simulink library "sphero_lib"  (Simulink 8.8)
settings: Solver=ode45  StartTime=0.0  StopTime=10.0  RelTol=1e-3
libraries: simulink x2
settings Model: Creator=gvallabh  LastModifiedBy=gcampa

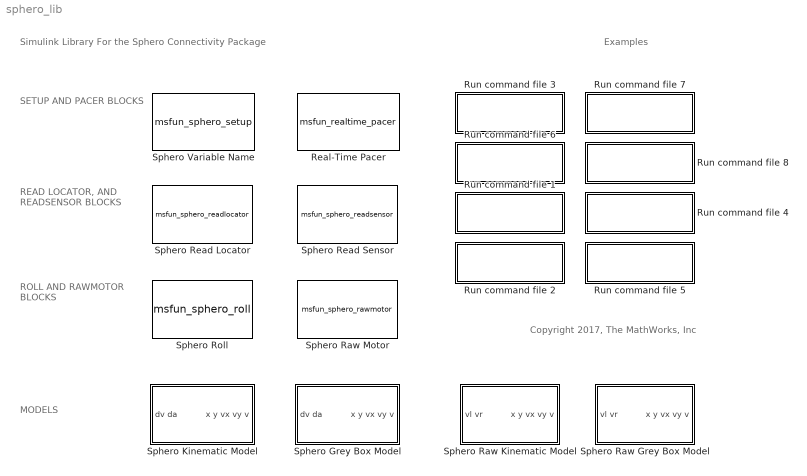
== system sphero_lib ==
  note: Copyright 2017, The MathWorks, Inc
  note: SETUP
      | AND PACER
      | BLOCKS
  note: Simulink Library For the Sphero Connectivity Package
  note: READ LOCATOR,
      | AND READSENSOR
      | BLOCKS
  note: Examples
  note: ROLL AND
      | RAWMOTOR
      | BLOCKS
  note: MODELS
  Real-Time Pacer : M-S-Function  FunctionName=msfun_realtime_pacer  Parameters=simTimePerRealTime  mask(RealTime_Pacer){simTimePerRealTime=1}
      mask prompts: simTimePerRealTime "Speedup (Simulation Time / Real Time):"
      mask help:
      | Slow down a simulation to track real (i.e., wall clock) elapsed time.
      |
      | "Speedup" specifies the ratio between simulation time and real time
      |  Speedup = N => N sec. of simulation time per sec. of real time
      |  Speedup can be fractional (e.g., 0.5, 1.3).
      |  Speedup = inf => allow simulation to run at full speed
      |
      | Click on the Help button for details.
      mask Help: web('realtime_pacer_help.html', '-helpbrowser')
      mask Display: fprintf('Real-Time Pacer\nSpeedup = %g', simTimePerRealTime)
  Run command file 1 : Subsystem
      settings: OpenFcn=rawmotor_sim
      mask Display: disp('Command \nRaw Motors')
  Run command file 2 : Subsystem
      settings: OpenFcn=sph_control_sim
      mask Display: disp('Control \nExample')
  Run command file 3 : Subsystem
      settings: OpenFcn=accel_sim
      mask Display: disp('Read Sensor \n (Acceleration)')
  Run command file 4 : Subsystem
      settings: OpenFcn=rawmotor_sim_kine
      mask Display: disp('Raw Kinematic Model\n Open Loop')
  Run command file 5 : Subsystem
      settings: OpenFcn=rawmotor_sim_grey
      mask Display: disp('Raw Grey Box Model\n Open Loop')
  Run command file 6 : Subsystem
      settings: OpenFcn=roll_sim
      mask Display: disp('Roll and\n Read Location')
  Run command file 7 : Subsystem
      settings: OpenFcn=sph_control_sim_kine
      mask Display: disp('Kinematic Model\n Control')
  Run command file 8 : Subsystem
      settings: OpenFcn=sph_control_sim_grey
      mask Display: disp('Grey Box Model\n Control')
  Sphero Grey Box Model : Subsystem  mask(Sphero Grey Box Model){num=[5.4], den=[1 3.8], vtr=[5 50], vmax=1500, Nva=[1 0.1], D=[1 1], P0=[0 0], T=0.1}
      mask prompts: num "Speed transfer function numerator"; den "Speed transfer function denominator"; vtr "Thresholds for current and desired speed (0 to 255)"; vmax "Maximum speed (mm/s)"; Nva "Input noise powers for desired speed and angle"; D "Send and Receive delay lengths"; P0 "Initial Position along x and y (cm)"; T "Sample Time"
      mask help:
      | This block is a grey-box model of the Sphero. The input vector contains the desired speed dv (from 0 to 255) and desired angle da in degrees. The output vector contains 5 elements: the positions along x and y axis (in mm), the velocities along the same axis (in mm/sec), and the total speed, (that is the magnitude of the velocity vector).
      |
      | The kinematics are modeled as an unicycle, that is [xdot ydot]=v*[sin(a) cos(a)] where v and a are speed and angle. The angle a is assumed equal to the desired angle input.
      |
      | The relationship between the speed v and the desired speed input dv is modeled by a continuous time transfer function (active when both the current and desired speed are greater than a given threshold), followed by a rescaling to the range [0 vmax], where vmax is the maximum speed (when dv=255) in mm/s. Noise is inserted at the block input, while transmission delays are used both at the block input and output.
      mask init:
      | x0=P0(1);y0=P0(2);
      mask Help:
      | This block is a grey-box model of the Sphero. The input vector contains the desired speed dv (from 0 to 255) and desired angle da in degrees. The output vector contains 5 elements: the positions along x and y axis (in mm), the velocities along the same axis (in mm/sec), and the total speed, (that is the magnitude of the velocity vector).
      | 
      | The kinematics are modeled as an unicycle, that is [xdot ydot]=v*[sin(a) cos(a)] where v and a are speed and angle. The angle a is assumed equal to the desired angle input.
      | 
      | The relationship between the speed v and the desired speed input dv is modeled by a continuous time transfer function (active when both the current and desired speed are greater than a given threshold), followed by a rescaling to the range [0 vmax], where vmax is the maximum speed (when dv=255) in mm/s. Noise is inserted at the block input, while transmission delays are used both at the block input and output.
      | 
      | Look under the mask for more information.
  Sphero Kinematic Model : Subsystem  mask(Sphero Kinematic Model){vmax=1500, P0=[0 0]}
      mask prompts: vmax "Max Speed (mm/s)"; P0 "Initial Position along x and y (cm)"
      mask help:
      | This block is a pure kinematic model of the Sphero.
      |
      | The input vector contains the desired speed dv (from 0 to 255) and desired angle da in degrees. The output vector contains 5 elements: the positions along x and y axis (in mm), the velocities along the same axis (in mm/sec), and the total speed, (that is the magnitude of the velocity vector).
      |
      | The kinematics are modeled as an unicycle, that is [xdot ydot]=v*[sin(a) cos(a)] where v and a are speed and angle. The angle a is assumed equal to the desired angle input da. The speed v is a rescaling of the input dv from the range [0 255] to the range [0 vmax],  (that is v=vmax/255*dv) where vmax is the maximum speed in mm/s.
      mask init:
      | x0=P0(1);y0=P0(2);
      mask Help:
      | This block is a pure kinematic model of the Sphero.
      | 
      | The input vector contains the desired speed dv (from 0 to 255) and desired angle da in degrees. The output vector contains 5 elements: the positions along x and y axis (in mm), the velocities along the same axis (in mm/sec), and the total speed, (that is the magnitude of the velocity vector).
      | 
      | The kinematics are modeled as an unicycle, that is [xdot ydot]=v*[sin(a) cos(a)] where v and a are speed and angle. The angle a is assumed equal to the desired angle input da. The speed v is a rescaling of the input dv from the range [0 255] to the range [0 vmax],  (that is v=vmax/255*dv) where vmax is the maximum speed in mm/s.
      | 
      | Please look under the mask for further information.
  Sphero Raw Grey Box Model : Subsystem  mask(Sphero Grey Box Model){num_v=[5.4], den_v=[1 3.8], vtr=[5 50], num_w=[0.59], den_w=[1 0.1], vmax=1500, Nvw=[1 0.1]*0, D=[1 1], T=0.1, P0=[0 0]}
      mask prompts: num_v "Speed transfer function numerator"; den_v "Speed transfer function denominator"; vtr "Thresholds for current and desired speed (0 to 255)"; num_w "Angular speed transfer function numerator"; den_w "Angular speed transfer function denominator"; vmax "Maximum speed (mm/s)"; Nvw "Input noise powers for desired speed and angle"; D "Send and Receive delay lengths"; T "Sample Time"; P0 "Initial Position along x and y (cm)"
      mask help:
      | This block is a grey-box model of the Sphero. The input vector contains the desired speed of left and right motors (from 0 to 255). The output vector contains 5 elements: the positions along x and y axis (in mm), the velocities along the same axis (in mm/sec), and the total speed, (that is the magnitude of the velocity vector).
      |
      | The kinematics are modeled as an unicycle, that is [xdot ydot]=v*[sin(a) cos(a)] where v and a are speed and angle. The relationship between the speed v and the speed command (L+R)/2  is modeled by a continuous time transfer function (active when both the current and desired speed are greater than a given threshold), followed by a rescaling to the range [0 vmax], where vmax is the maximum speed (when dv=255) in mm/s. The  relationship between the angle a and the angular speed command (L-R)/2  is modeled by a continuous time transfer function (having static gain equal to wmax/255, where wmax is the maximum angular speed) followed by an integrator. Noise is inserted at the block input, while transmission delays are used both at the block input and output.
      mask init:
      | x0=P0(1);y0=P0(2);
      mask Help:
      | This block is a grey-box model of the Sphero. The input vector contains the desired speed of left and right motors (from 0 to 255). The output vector contains 5 elements: the positions along x and y axis (in mm), the velocities along the same axis (in mm/sec), and the total speed, (that is the magnitude of the velocity vector).
      | 
      | The kinematics are modeled as an unicycle, that is [xdot ydot]=v*[sin(a) cos(a)] where v and a are speed and angle. The relationship between the speed v and the speed command (L+R)/2  is modeled by a continuous time transfer function (active when both the current and desired speed are greater than a given threshold), followed by a rescaling to the range [0 vmax], where vmax is the maximum speed (when dv=255) in mm/s. The  relationship between the angle a and the angular speed command (L-R)/2  is modeled by a continuous time transfer function (having static gain equal to wmax/255, where wmax is the maximum angular speed) followed by an integrator. Noise is inserted at the block input, while transmission delays are used both at the block input and output.
      | 
      | Look under the mask for more information.
  "Sphero Raw Kinematic Model " : Subsystem  mask(Sphero Grey Box Model){vmax=1500, wmax=1500, P0=[0 0]}
      mask prompts: vmax "Maximum speed (mm/s)"; wmax "Maximum angular speed (deg/s)"; P0 "Initial Position along x and y (cm)"
      mask help:
      | This block is a grey-box model of the Sphero. The input vector contains the desired speed of left and right motors (from 0 to 255). The output vector contains 5 elements: the positions along x and y axis (in mm), the velocities along the same axis (in mm/sec), and the total speed, (that is the magnitude of the velocity vector).
      |
      | The kinematics are modeled as an unicycle, that is [xdot ydot]=v*[sin(a) cos(a)] where v and a are speed and angle. The speed v is a rescaling of the the speed input (L+R)/2 from the range [0 255] to the range [0 vmax],  (that is v=vmax/255*(L+R)/2) where vmax is the maximum speed in mm/s. Similarly, the angluar speed w is a rescaling of the the anngular speed input (L-R)/2 from the range [0 255] to the range [0 wmax],  (that is v=wmax/255*(L-R)/2) where wmax is the maximum angular speed in deg/s. The angle a is the integral of the angular speed.
      mask init:
      | x0=P0(1);y0=P0(2);
      mask Help:
      | This block is a grey-box model of the Sphero. The input vector contains the desired speed of left and right motors (from 0 to 255). The output vector contains 5 elements: the positions along x and y axis (in mm), the velocities along the same axis (in mm/sec), and the total speed, (that is the magnitude of the velocity vector).
      | 
      | The kinematics are modeled as an unicycle, that is [xdot ydot]=v*[sin(a) cos(a)] where v and a are speed and angle. The speed v is a rescaling of the the speed input (L+R)/2 from the range [0 255] to the range [0 vmax],  (that is v=vmax/255*(L+R)/2) where vmax is the maximum speed in mm/s. Similarly, the angluar speed w is a rescaling of the the anngular speed input (L-R)/2 from the range [0 255] to the range [0 wmax],  (that is v=wmax/255*(L-R)/2) where wmax is the maximum angular speed in deg/s. The angle a is the integral of the angular speed.
      | 
      | Look under the mask for more information.
  Sphero Raw Motor : M-S-Function  FunctionName=msfun_sphero_rawmotor  Parameters="SpheroVarNumber,  T"  mask(Sphero Raw Motor){SpheroVarNumber=Existing workspace Sphero variable #1, T=0.2}
      mask prompts: SpheroVarNumber "Sphero Variable"; T "Sample Time (-1 for inherited)"
      mask help:
      | Every time this block is executed it gets the 2-elements vector at its input, which contains the power of the left and right motors respectively, and calls the MATLAB "rawMotor" function to move the Sphero motors accordingly. Note that the mode is set to reverse if the specified speed is negative.
      |
      | The first parameter in the mask is the name of the Sphero object (which must match the one chosen in the Setup block). The second parameter is the sample time.
      |
      | See the help for more details.
      mask Help:
      | Every time this block is executed it gets the 2-elements vector at its input, which contains the power of the left and right motors respectively, and calls the MATLAB "rawMotor" function to move the Sphero motors accordingly. Note that the mode is set to reverse if the specified speed is negative.
      | 
      | The first parameter in the mask is the name of the Sphero object (which must match the one chosen in the Setup block). The second parameter is the sample time.
      | 
      | The corresponding Sphero method is "rawMotor", so you can type "doc sphero.rawMotor" or "help sphero.rawMotor" for more details.
      mask TypeOptions SpheroVarNumber: Existing workspace Sphero variable #1 | Existing workspace Sphero variable #2 | Existing workspace Sphero variable #3 | Existing workspace Sphero variable #4
      mask Display:
      | try
      |     SetupBlockName = find_system(bdroot(gcb),'SearchDepth', 1, 'MaskType', 'Sphero Name Setup', 'SpheroVarNumber', SpheroVarNumber);
      |     str=get_param(SetupBlockName,'workspaceVarName');
      |     fprintf('%s\nrawMotor\n',str{1});
      | catch
      |     fprintf('Workspace var #%s\nrawMotor\n',SpheroVarNumber(end))
      | end
      | 
      | color('gray')
      | fprintf('\n\n [left right]');
  Sphero Read Locator : M-S-Function  FunctionName=msfun_sphero_readlocator  Parameters=SpheroVarNumber, T  mask(Sphero Read Locator){SpheroVarNumber=Existing workspace Sphero variable #1, T=0.2}
      mask prompts: SpheroVarNumber "Sphero Variable"; T "Sample Time (-1 for inherited):"
      mask help:
      | Every time this block is executed it calls the MATLAB "readLocator" function, which returns the current location and velocity components of the Sphero.
      |
      | The output of the block is a 5-element vector containing respectively the position along the x and y axes, the velocity along x and y axes, and the speed of the Sphero.
      |
      | The first parameter in the mask is the name of the Sphero object (which must match the one chosen in the Setup block).
      | The second parameter is the sample time.
      |
      | See the help for more details.
      mask Help:
      | Every time this block is executed it calls the MATLAB readLocator function, which returns the current location and velocity components of the Sphero.
      | 
      | The output of the block is a 5-element vector containing respectively the position along the x and y axes, the velocity along x and y axes, and the speed of the Sphero.
      | 
      | All the data received from the sphero are int16 values, which are then casted to doubles at the block output. Specifically, the positions are signed values in cm, velocities are signed in cm/sec, and the speed is unsigned in cm/sec.
      | 
      | The first parameter in the mask is the name of the Sphero object (which must match the one chosen in the Setup block).
      | The second parameter is the sample time.
      | 
      | The corresponding MATLAB command is "readLocator", so you can type "doc sphero.readLocator" or "help sphero.readLocator" for more details.
      mask TypeOptions SpheroVarNumber: Existing workspace Sphero variable #1 | Existing workspace Sphero variable #2 | Existing workspace Sphero variable #3 | Existing workspace Sphero variable #4
      mask Display:
      | try
      |     SetupBlockName = find_system(bdroot(gcb),'SearchDepth', 1, 'MaskType', 'Sphero Name Setup', 'SpheroVarNumber', SpheroVarNumber);
      |     str=get_param(SetupBlockName,'workspaceVarName');
      |     fprintf('%s\nreadLocator\n',str{1});
      | catch
      |     fprintf('Workspace var #%s\nreadLocator\n',SpheroVarNumber(end))
      | end
      | 
      | color('gray')
      | fprintf('\n\n [x  y  vx  vy  v]');
  Sphero Read Sensor : M-S-Function  FunctionName=msfun_sphero_readsensor  Parameters=SpheroVarNumber, SensorString, T  mask(Sphero Read Sensor){SpheroVarNumber=Existing workspace Sphero variable #1, SensorString=accelX, T=1}
      mask prompts: SpheroVarNumber "Sphero Variable"; SensorString "Sensor"; T "Sample Time (-1 for inherited):"
      mask help:
      | Every time this block is executed it calls the MATLAB "readSensor" function, which reads a specified sensor and returns its value.
      |
      | The output of the block is a scalar containing the value measured by the sensor.
      |
      | The first parameter in the mask is the name of the Sphero object (which must match the one chosen in the Setup block).
      | The second parameter is the sensor to be read.
      | The third parameter is the sample time.
      |
      | See the help for more details.
      mask Help:
      | Every time this block is executed it calls the MATLAB "readSensor" function, which reads a specified sensor and returns its value.
      | 
      | The output of the block is a scalar containing the value measured by the sensor.
      | All the data received from the sphero are int16 values, which are then casted to doubles at the block output. Specifically, the positions are signed values in cm, velocities are signed in cm/sec, and the speed is unsigned in cm/sec.
      | 
      | The first parameter in the mask is the name of the Sphero object (which must match the one chosen in the Setup block).
      | 
      | The second parameter is the sensor to be read.It must be one of these strings: 'accelX', 'accelY', 'accelZ', 'gyroX', 'gyroY', 'gyroZ','rmotorEmfRaw', 'lmotorEmfRaw', 'lmotorPwmRaw', 'rmotorPwmRaw','imuPitch', 'imuRoll', 'imuYaw', 'accelXFilt', 'accelYFilt','accelZFilt', 'gyroXFilt', 'gyroYFilt', 'gyroZFilt','rmotorEmfFilt', 'lmotorEmfFilt', 'Q0', 'Q1', 'Q2', 'Q3', 'distX','distY', 'accelOne', 'velX', 'velY'
      | 
      | The third parameter is the sample time.
      mask TypeOptions SpheroVarNumber: Existing workspace Sphero variable #1 | Existing workspace Sphero variable #2 | Existing workspace Sphero variable #3 | Existing workspace Sphero variable #4
      mask TypeOptions SensorString: accelX | accelY | accelZ | gyroX | gyroY | gyroZ | rmotorEmfRaw  | lmotorEmfRaw | lmotorPwmRaw  | rmotorPwmRaw | imuPitch | imuRoll | imuYaw | accelXFilt | accelYFilt | accelZFilt | gyroXFilt | gyroYFilt | gyroZFilt | rmotorEmfFilt | lmotorEmfFilt | Q0 | Q1 | Q2 | Q3 | distX | distY | accelOne | velX  | velY
      mask Display:
      | try
      |     SetupBlockName = find_system(bdroot(gcb),'SearchDepth', 1, 'MaskType', 'Sphero Name Setup', 'SpheroVarNumber', SpheroVarNumber);
      |     str=get_param(SetupBlockName,'workspaceVarName');
      |     fprintf('%s\nreadSensor\n',str{1});
      | catch
      |     fprintf('Workspace var #%s\nreadSensor\n',SpheroVarNumber(end))
      | end
      | 
      | sns=get_param(gcb,'SensorString');
      | color('gray')
      | fprintf('\n\n %s',sns);
  Sphero Roll : M-S-Function  FunctionName=msfun_sphero_roll  Parameters="SpheroVarNumber,  T"  mask(Sphero Roll){SpheroVarNumber=Existing workspace Sphero variable #1, T=0.2}
      mask prompts: SpheroVarNumber "Sphero Variable"; T "Sample Time (-1 for inherited)"
      mask help:
      | Every time this block is executed it gets the 2-elements vector at its input, which contains the desired speed ane heading for the Sphero, and calls the MATLAB "roll" function to move the Sphero accordingly.
      |
      | The first parameter in the mask is the name of the Sphero object (which must match the one chosen in the Setup block). The second parameter is the sample time.
      |
      | See the help for more details.
      mask Help:
      | Every time this block is executed it gets the 2-elements vector at its input, which contains the desired speed ane heading for the Sphero, and calls the MATLAB "roll" function to move the Sphero accordingly.
      | 
      | The first parameter in the mask is the name of the Sphero object (which must match the one chosen in the Setup block). The second parameter is the sample time.
      | 
      | The heading is a value from 0 to 360, which is specified with regards to the original orientation that is set when the Sphero is first connected, or calibrated to. Speed can be between -255 and 255
      | 
      | The corresponding Sphero method is "roll", so you can type "doc sphero.roll" or "help sphero.roll" for more details.
      mask TypeOptions SpheroVarNumber: Existing workspace Sphero variable #1 | Existing workspace Sphero variable #2 | Existing workspace Sphero variable #3 | Existing workspace Sphero variable #4
      mask Display:
      | try
      |     SetupBlockName = find_system(bdroot(gcb),'SearchDepth', 1, 'MaskType', 'Sphero Name Setup', 'SpheroVarNumber', SpheroVarNumber);
      |     str=get_param(SetupBlockName,'workspaceVarName');
      |     fprintf('%s\nroll\n',str{1});
      | catch
      |     fprintf('Workspace var #%s\nroll\n',SpheroVarNumber(end))
      | end
      | 
      | color('gray')
      | fprintf('\n\n [speed heading]');
  Sphero Variable Name : M-S-Function  Priority=3  FunctionName=msfun_sphero_setup  Parameters=SpheroVarNumber, workspaceVarName  mask(Sphero Name Setup){SpheroVarNumber=Existing workspace Sphero variable #1, workspaceVarName=sph}
      mask prompts: SpheroVarNumber "Sphero variable"; workspaceVarName "Name of existing workspace variable"
      mask help: An existing workspace Sphero variable must be selected as the mask parameter. That preexisitng Sphero object is then used during the simulation by the other blocks that specify the same name. The object will continue to be available in the workspace after the end of the simulation.
      mask Help: An existing workspace Sphero variable must be selected as the mask parameter. That preexisitng Sphero object is then used during the simulation by the other blocks that specify the same name. The object will continue to be available in the workspace after the end of the simulation.
      mask TypeOptions SpheroVarNumber: Existing workspace Sphero variable #1 | Existing workspace Sphero variable #2 | Existing workspace Sphero variable #3 | Existing workspace Sphero variable #4
      mask Display:
      | try
      |     BluetoothName=evalin('base',[workspaceVarName '.DeviceName']);
      | catch
      |     BluetoothName='Unknown';
      | end
      | fprintf('Setup\n%s\n%s',workspaceVarName, BluetoothName)

== system sphero_lib/Run command file 1 ==

== system sphero_lib/Run command file 2 ==

== system sphero_lib/Run command file 3 ==

== system sphero_lib/Run command file 4 ==

== system sphero_lib/Run command file 5 ==

== system sphero_lib/Run command file 6 ==

== system sphero_lib/Run command file 7 ==

== system sphero_lib/Run command file 8 ==

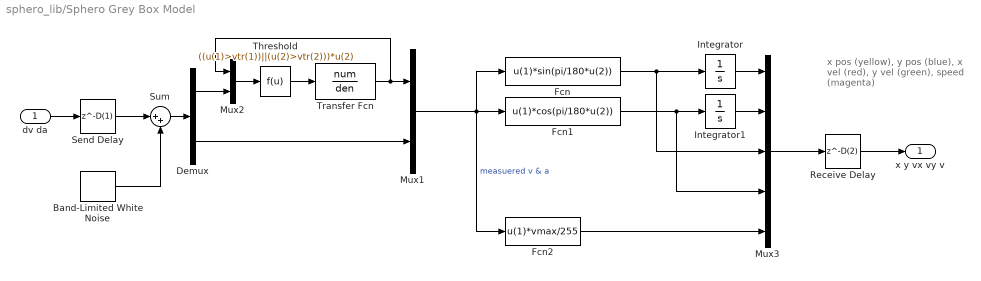
== system sphero_lib/Sphero Grey Box Model ==
  note: x pos (yellow),
      | y pos (blue),
      | x vel (red),
      | y vel (green),
      | speed (magenta)
  dv da : Inport
  Band-Limited White Noise : simulink/Sources/Band-Limited White Noise  Cov=Nva  Ts=T  seed=[1 2]
  Demux : Demux  Outputs=2
  Fcn : Fcn  Expr=u(1)*sin(pi/180*u(2))
  Fcn1 : Fcn  Expr=u(1)*cos(pi/180*u(2))
  Fcn2 : Fcn  Expr=u(1)*vmax/255
  Integrator : Integrator  InitialCondition=double(x0)
  Integrator1 : Integrator  InitialCondition=double(y0)
  Mux1 : Mux  Inputs=2
  Mux2 : Mux  Inputs=2
  Mux3 : Mux  Inputs=5
  Receive Delay : Delay  DelayLength=D(2)  SampleTime=T
  Send Delay : Delay  DelayLength=D(1)  SampleTime=T
  Sum : Sum  Inputs=|++
  Threshold : Fcn  Expr=((u(1)>vtr(1))||(u(2)>vtr(2)))*u(2)
  Transfer Fcn : TransferFcn  Numerator=num  Denominator=den
  x y vx vy v : Outport
  wires:
  Demux/1 -> Mux2/2
  Mux2/1 -> Threshold/1
  Sum/1 -> Demux/1
  Band-Limited White Noise/1 -> Sum/2
  Send Delay/1 -> Sum/1
  Demux/2 -> Mux1/2
  Threshold/1 -> Transfer Fcn/1
  Transfer Fcn/1 -> Mux1/1, Mux2/1
  Mux1/1 -> Fcn1/1, Fcn/1, Fcn2/1  "measuered v & a"
  Receive Delay/1 -> x y vx vy v/1
  Fcn2/1 -> Mux3/5
  Fcn1/1 -> Integrator1/1, Mux3/4
  Mux3/1 -> Receive Delay/1
  dv da/1 -> Send Delay/1
  Fcn/1 -> Integrator/1, Mux3/3
  Integrator/1 -> Mux3/1
  Integrator1/1 -> Mux3/2

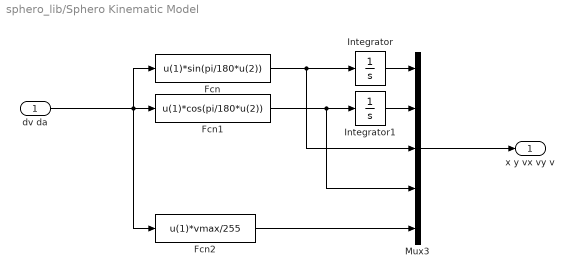
== system sphero_lib/Sphero Kinematic Model ==
  dv da : Inport
  Fcn : Fcn  Expr=u(1)*sin(pi/180*u(2))
  Fcn1 : Fcn  Expr=u(1)*cos(pi/180*u(2))
  Fcn2 : Fcn  Expr=u(1)*vmax/255
  Integrator : Integrator  InitialCondition=double(x0)
  Integrator1 : Integrator  InitialCondition=double(y0)
  Mux3 : Mux  Inputs=5
  x y vx vy v : Outport
  wires:
  Fcn2/1 -> Mux3/5
  Fcn1/1 -> Integrator1/1, Mux3/4
  Mux3/1 -> x y vx vy v/1
  dv da/1 -> Fcn1/1, Fcn/1, Fcn2/1
  Fcn/1 -> Integrator/1, Mux3/3
  Integrator/1 -> Mux3/1
  Integrator1/1 -> Mux3/2

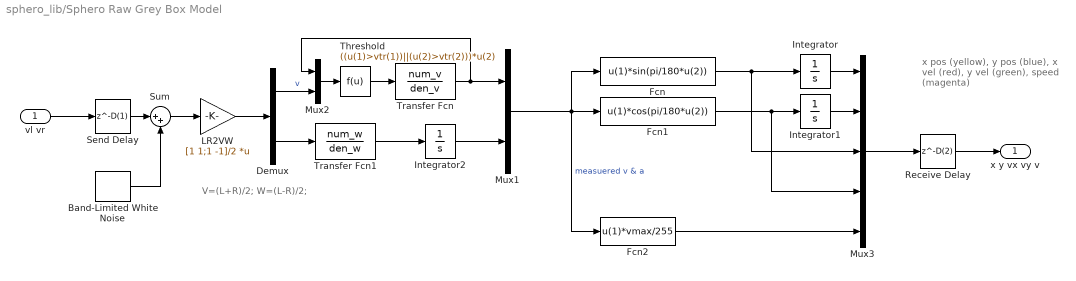
== system sphero_lib/Sphero Raw Grey Box Model ==
  note: x pos (yellow),
      | y pos (blue),
      | x vel (red),
      | y vel (green),
      | speed (magenta)
  note: V=(L+R)/2;
      | W=(L-R)/2;
  "vl vr " : Inport
  Band-Limited White Noise : simulink/Sources/Band-Limited White Noise  Cov=Nvw  Ts=T  seed=[1 2]
  Demux : Demux  Outputs=2
  Fcn : Fcn  Expr=u(1)*sin(pi/180*u(2))
  Fcn1 : Fcn  Expr=u(1)*cos(pi/180*u(2))
  Fcn2 : Fcn  Expr=u(1)*vmax/255
  Integrator : Integrator  InitialCondition=double(x0)
  Integrator1 : Integrator  InitialCondition=double(y0)
  Integrator2 : Integrator
  LR2VW : Gain  Gain=[1 1;1 -1]/2  Multiplication=Matrix(K*u)
  Mux1 : Mux  Inputs=2
  Mux2 : Mux  Inputs=2
  Mux3 : Mux  Inputs=5
  Receive Delay : Delay  DelayLength=D(2)  SampleTime=T
  Send Delay : Delay  DelayLength=D(1)  SampleTime=T
  Sum : Sum  Inputs=|++
  Threshold : Fcn  Expr=((u(1)>vtr(1))||(u(2)>vtr(2)))*u(2)
  Transfer Fcn : TransferFcn  Numerator=num_v  Denominator=den_v
  Transfer Fcn1 : TransferFcn  Numerator=num_w  Denominator=den_w
  x y vx vy v : Outport
  wires:
  "vl vr "/1 -> Send Delay/1
  Integrator1/1 -> Mux3/2
  Integrator/1 -> Mux3/1
  Fcn/1 -> Mux3/3, Integrator/1
  Mux3/1 -> Receive Delay/1
  Fcn1/1 -> Mux3/4, Integrator1/1
  Fcn2/1 -> Mux3/5
  Receive Delay/1 -> x y vx vy v/1
  Mux1/1 -> Fcn2/1, Fcn/1, Fcn1/1  "measuered v & a"
  Transfer Fcn/1 -> Mux2/1, Mux1/1
  Threshold/1 -> Transfer Fcn/1
  Demux/2 -> Transfer Fcn1/1
  Send Delay/1 -> Sum/1
  Band-Limited White Noise/1 -> Sum/2
  Sum/1 -> LR2VW/1
  Mux2/1 -> Threshold/1
  Demux/1 -> Mux2/2  "v"
  LR2VW/1 -> Demux/1
  Integrator2/1 -> Mux1/2
  Transfer Fcn1/1 -> Integrator2/1

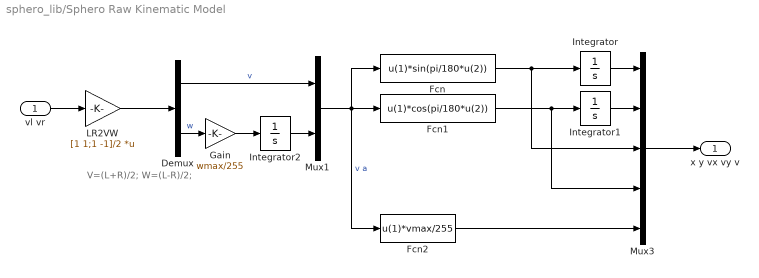
== system sphero_lib/Sphero Raw Kinematic Model  ==
  note: V=(L+R)/2;
      | W=(L-R)/2;
  "vl vr " : Inport
  Demux : Demux  Outputs=2
  Fcn : Fcn  Expr=u(1)*sin(pi/180*u(2))
  Fcn1 : Fcn  Expr=u(1)*cos(pi/180*u(2))
  Fcn2 : Fcn  Expr=u(1)*vmax/255
  Gain : Gain  Gain=wmax/255
  Integrator : Integrator  InitialCondition=double(x0)
  Integrator1 : Integrator  InitialCondition=double(y0)
  Integrator2 : Integrator  InitialCondition=double(x0)
  LR2VW : Gain  Gain=[1 1;1 -1]/2  Multiplication=Matrix(K*u)
  Mux1 : Mux  Inputs=2
  Mux3 : Mux  Inputs=5
  x y vx vy v : Outport
  wires:
  Integrator1/1 -> Mux3/2
  Integrator/1 -> Mux3/1
  Fcn/1 -> Mux3/3, Integrator/1
  Fcn1/1 -> Mux3/4, Integrator1/1
  Fcn2/1 -> Mux3/5
  Mux3/1 -> x y vx vy v/1
  Mux1/1 -> Fcn2/1, Fcn/1, Fcn1/1  "v a"
  LR2VW/1 -> Demux/1
  Integrator2/1 -> Mux1/2
  Demux/2 -> Gain/1  "w"
  Demux/1 -> Mux1/1  "v"
  Gain/1 -> Integrator2/1
  "vl vr "/1 -> LR2VW/1
